simulink model "blockdemo"  (Simulink 7.0)
settings: Solver=VariableStepDiscrete  StartTime=0.0  StopTime=20  FixedStep=1  RelTol=1e-3
InitFcn:
  | %% DSPBuilder Start
  | alt_dspbuilder_update_model(bdroot)
  | %% DSPBuilder End
libraries: allblocks_alteradspbuilder2 x19
settings Model: Creator=mjervis  LastModifiedBy=delphick
settings OptimizationCC: BlockReduction=off  BooleanDataType=off  InlineInvariantSignals=on
settings DebuggingCC: SaveWithParameterizedLinksMsg=none  SignalResolutionControl=TryResolveAllWithWarning  SolverPrmCheckMsg=none  MultiTaskDSMMsg=warning  MultiTaskCondExecSysMsg=none
settings HardwareCC: TargetUnknown=on
settings RTWCC: IncludeERTFirstTime=on
settings GRTTargetCC: TargetFcnLib=ansi_tfl_tmw.mat

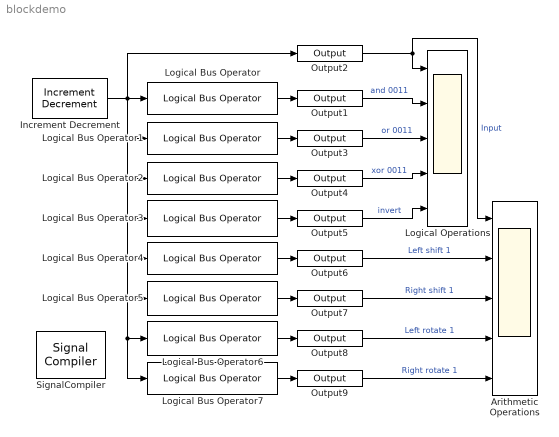
== system blockdemo ==
  Arithmetic Operations : Scope  NumInputPorts=5
      settings: TimeRange=20  YMin=0~0~0~0~0  YMax=20~20~10~20~20
  Increment Decrement : allblocks_alteradspbuilder2/Increment Decrement  BusType=Unsigned Integer  bwl=4  bwr=0  SpecifyClock=off  clr_value=0  direction=Increment  phase_selection=1  use_ena=off  use_sclr=off  pipeline_display=1
  Logical Bus Operator : allblocks_alteradspbuilder2/Logical Bus Operator  BusType=Unsigned Integer  bwl=4  bwr=0  LogicalOp_text=AND  mask_value_num=3  shift_amount=0  force_sign_ext=off  pipeline_display=0
  Logical Bus Operator1 : allblocks_alteradspbuilder2/Logical Bus Operator  BusType=Unsigned Integer  bwl=4  bwr=0  LogicalOp_text=OR  mask_value_num=3  shift_amount=0  force_sign_ext=off  pipeline_display=0
  Logical Bus Operator2 : allblocks_alteradspbuilder2/Logical Bus Operator  BusType=Unsigned Integer  bwl=4  bwr=0  LogicalOp_text=XOR  mask_value_num=3  shift_amount=0  force_sign_ext=off  pipeline_display=0
  Logical Bus Operator3 : allblocks_alteradspbuilder2/Logical Bus Operator  BusType=Unsigned Integer  bwl=4  bwr=0  LogicalOp_text=Invert  mask_value_num=3  shift_amount=0  force_sign_ext=off  pipeline_display=0
  Logical Bus Operator4 : allblocks_alteradspbuilder2/Logical Bus Operator  BusType=Unsigned Integer  bwl=4  bwr=0  LogicalOp_text=Shift Left  mask_value_num=3  shift_amount=1  force_sign_ext=off  pipeline_display=0
  Logical Bus Operator5 : allblocks_alteradspbuilder2/Logical Bus Operator  BusType=Signed Integer  bwl=4  bwr=0  LogicalOp_text=Shift Right  mask_value_num=3  shift_amount=1  force_sign_ext=off  pipeline_display=0
  Logical Bus Operator6 : allblocks_alteradspbuilder2/Logical Bus Operator  BusType=Unsigned Integer  bwl=4  bwr=0  LogicalOp_text=Rotate Left  mask_value_num=3  shift_amount=1  force_sign_ext=off  pipeline_display=0
  Logical Bus Operator7 : allblocks_alteradspbuilder2/Logical Bus Operator  BusType=Unsigned Integer  bwl=4  bwr=0  LogicalOp_text=Rotate Right  mask_value_num=3  shift_amount=1  force_sign_ext=off  pipeline_display=0
  Logical Operations : Scope  NumInputPorts=5
      settings: TimeRange=20  YMin=0~0~0~0~0  YMax=20~4~20~20~20
  Output1 : allblocks_alteradspbuilder2/Output  iofile=C:\perforce_workspace81\main\dsp_builder2\Documentation\DesignExamples\Tutorials\UnitBlocks\GateAndControl\LogicalBusOperator\tb_blockdemo\blockdemo_Output1.capture  BusType=Inferred  bwl=4  bwr=0  externalType=Inferred  PORTTYPE=Output  allowFloatingPointOverride=on  logOutputs=off
  Output2 : allblocks_alteradspbuilder2/Output  iofile=C:\perforce_workspace81\main\dsp_builder2\Documentation\DesignExamples\Tutorials\UnitBlocks\GateAndControl\LogicalBusOperator\tb_blockdemo\blockdemo_Output2.capture  BusType=Inferred  bwl=4  bwr=0  externalType=Inferred  PORTTYPE=Output  allowFloatingPointOverride=on  logOutputs=off
  Output3 : allblocks_alteradspbuilder2/Output  iofile=C:\perforce_workspace81\main\dsp_builder2\Documentation\DesignExamples\Tutorials\UnitBlocks\GateAndControl\LogicalBusOperator\tb_blockdemo\blockdemo_Output3.capture  BusType=Inferred  bwl=4  bwr=0  externalType=Inferred  PORTTYPE=Output  allowFloatingPointOverride=on  logOutputs=off
  Output4 : allblocks_alteradspbuilder2/Output  iofile=C:\perforce_workspace81\main\dsp_builder2\Documentation\DesignExamples\Tutorials\UnitBlocks\GateAndControl\LogicalBusOperator\tb_blockdemo\blockdemo_Output4.capture  BusType=Inferred  bwl=4  bwr=0  externalType=Inferred  PORTTYPE=Output  allowFloatingPointOverride=on  logOutputs=off
  Output5 : allblocks_alteradspbuilder2/Output  iofile=C:\perforce_workspace81\main\dsp_builder2\Documentation\DesignExamples\Tutorials\UnitBlocks\GateAndControl\LogicalBusOperator\tb_blockdemo\blockdemo_Output5.capture  BusType=Inferred  bwl=4  bwr=0  externalType=Inferred  PORTTYPE=Output  allowFloatingPointOverride=on  logOutputs=off
  Output6 : allblocks_alteradspbuilder2/Output  iofile=C:\perforce_workspace81\main\dsp_builder2\Documentation\DesignExamples\Tutorials\UnitBlocks\GateAndControl\LogicalBusOperator\tb_blockdemo\blockdemo_Output6.capture  BusType=Inferred  bwl=4  bwr=0  externalType=Inferred  PORTTYPE=Output  allowFloatingPointOverride=on  logOutputs=off
  Output7 : allblocks_alteradspbuilder2/Output  iofile=C:\perforce_workspace81\main\dsp_builder2\Documentation\DesignExamples\Tutorials\UnitBlocks\GateAndControl\LogicalBusOperator\tb_blockdemo\blockdemo_Output7.capture  BusType=Inferred  bwl=4  bwr=0  externalType=Inferred  PORTTYPE=Output  allowFloatingPointOverride=on  logOutputs=off
  Output8 : allblocks_alteradspbuilder2/Output  iofile=C:\perforce_workspace81\main\dsp_builder2\Documentation\DesignExamples\Tutorials\UnitBlocks\GateAndControl\LogicalBusOperator\tb_blockdemo\blockdemo_Output8.capture  BusType=Inferred  bwl=4  bwr=0  externalType=Inferred  PORTTYPE=Output  allowFloatingPointOverride=on  logOutputs=off
  Output9 : allblocks_alteradspbuilder2/Output  iofile=C:\perforce_workspace81\main\dsp_builder2\Documentation\DesignExamples\Tutorials\UnitBlocks\GateAndControl\LogicalBusOperator\tb_blockdemo\blockdemo_Output9.capture  BusType=Inferred  bwl=4  bwr=0  externalType=Inferred  PORTTYPE=Output  allowFloatingPointOverride=on  logOutputs=off
  SignalCompiler : allblocks_alteradspbuilder2/Signal Compiler  DeviceFamily=Stratix IV  DeviceName=AUTO  EnableSignalTap=off  SignalTapDepth=128  UseBoardBlock=off  StpUseDefaultClock=on  StpClock=Clock  ExportDir=C:\Documents and Settings\delphick\My Documents\MATLAB
  wires:
  Output1/1 -> Logical Operations/2  "and 0011"
  Increment Decrement/1 -> Logical Bus Operator/1, Output2/1, Logical Bus Operator1/1, Logical Bus Operator2/1, Logical Bus Operator3/1, Logical Bus Operator4/1, Logical Bus Operator5/1, Logical Bus Operator6/1, Logical Bus Operator7/1
  Logical Bus Operator/1 -> Output1/1
  Output2/1 -> Logical Operations/1, Arithmetic Operations/1  "Input"
  Output3/1 -> Logical Operations/3  "or 0011"
  Logical Bus Operator1/1 -> Output3/1
  Output4/1 -> Logical Operations/4  "xor 0011"
  Logical Bus Operator2/1 -> Output4/1
  Output5/1 -> Logical Operations/5  "invert"
  Logical Bus Operator3/1 -> Output5/1
  Output6/1 -> Arithmetic Operations/2  "Left shift 1"
  Logical Bus Operator4/1 -> Output6/1
  Output7/1 -> Arithmetic Operations/3  "Right shift 1"
  Logical Bus Operator5/1 -> Output7/1
  Output8/1 -> Arithmetic Operations/4  "Left rotate 1"
  Output9/1 -> Arithmetic Operations/5  "Right rotate 1"
  Logical Bus Operator7/1 -> Output9/1
  Logical Bus Operator6/1 -> Output8/1
